simulink model "triplestageSimu"  (R2015a)
settings: Solver=ode45  StartTime=0.0  StopTime=10.0  RelTol=1e-3
values from neighbouring files (symbols this model uses):
  b1 = 0.1    [measfreqresp.m]
  b2 = 0.2    [measfreqresp.m]
  b3 = 0.1    [measfreqresp.m]
  b4 = 0.1    [measfreqresp.m]
libraries: fl_lib x21, nesl_utility x7
settings Model: Creator=Jinwen  LastModifiedBy=Jinwen

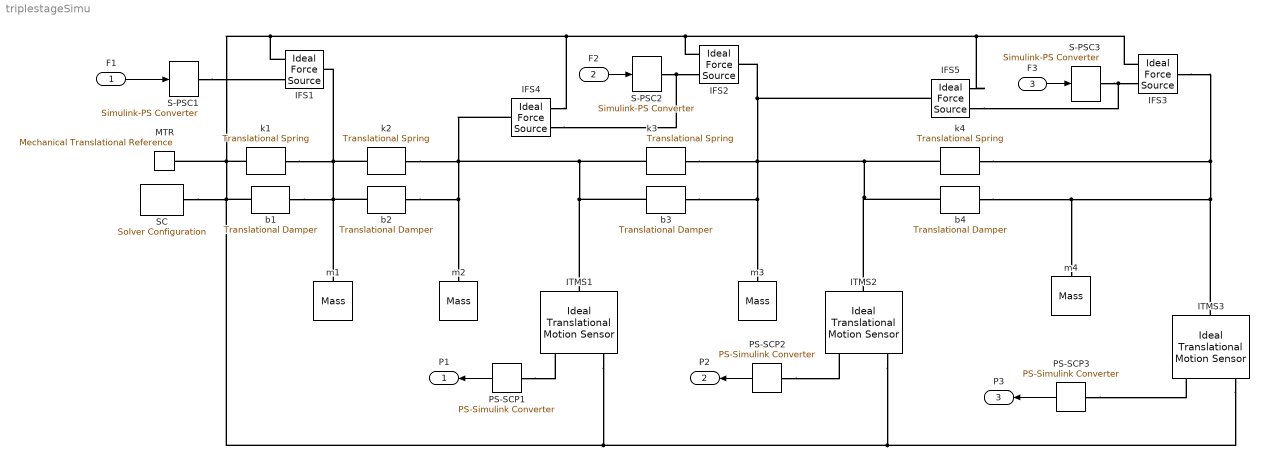
== system triplestageSimu ==
  F1 : Inport
  F2 : Inport  Port=2
  F3 : Inport  Port=3
  IFS{1..5} (5 alike) : fl_lib/Mechanical/Mechanical Sources/Ideal Force Source
  ITMS1 : fl_lib/Mechanical/Mechanical Sensors/Ideal Translational Motion Sensor  offset=0 m
  ITMS2 : fl_lib/Mechanical/Mechanical Sensors/Ideal Translational Motion Sensor  offset=0 m
  ITMS3 : fl_lib/Mechanical/Mechanical Sensors/Ideal Translational Motion Sensor  offset=0 m
  MTR : fl_lib/Mechanical/Translational Elements/Mechanical Translational Reference
  PS-SCP1 : nesl_utility/PS-Simulink Converter  PhysicalDomain=network_engine_domain  SubClassName=ps_output  LeftPortType=input  RightPortType=output  PseudoPeriodic=off  Frequencies=[]  Unit=1  AffineConversion=off
  PS-SCP2 : nesl_utility/PS-Simulink Converter  PhysicalDomain=network_engine_domain  SubClassName=ps_output  LeftPortType=input  RightPortType=output  PseudoPeriodic=off  Frequencies=[]  Unit=1  AffineConversion=off
  PS-SCP3 : nesl_utility/PS-Simulink Converter  PhysicalDomain=network_engine_domain  SubClassName=ps_output  LeftPortType=input  RightPortType=output  PseudoPeriodic=off  Frequencies=[]  Unit=1  AffineConversion=off
  S-PSC1 : nesl_utility/Simulink-PS Converter  PhysicalDomain=network_engine_domain  SubClassName=ps_input  LeftPortType=input  RightPortType=output  PseudoPeriodic=off  Frequencies=[]  NoiseDistribution=none  NoiseParameters=[]  Unit=1  AffineConversion=off  InputFiltering=off  SimscapeFilterOrder=1  InputFilterTimeConstant=0.001  UdotUserProvided=1
  S-PSC2 : nesl_utility/Simulink-PS Converter  PhysicalDomain=network_engine_domain  SubClassName=ps_input  LeftPortType=input  RightPortType=output  PseudoPeriodic=off  Frequencies=[]  NoiseDistribution=none  NoiseParameters=[]  Unit=1  AffineConversion=off  InputFiltering=off  SimscapeFilterOrder=1  InputFilterTimeConstant=0.001  UdotUserProvided=1
  S-PSC3 : nesl_utility/Simulink-PS Converter  PhysicalDomain=network_engine_domain  SubClassName=ps_input  LeftPortType=input  RightPortType=output  PseudoPeriodic=off  Frequencies=[]  NoiseDistribution=none  NoiseParameters=[]  Unit=1  AffineConversion=off  InputFiltering=off  SimscapeFilterOrder=1  InputFilterTimeConstant=0.001  UdotUserProvided=1
  SC : nesl_utility/Solver Configuration  PhysicalDomain=network_engine_domain  SubClassName=solver  LeftPortType=input  RightPortType=generic  Accelerate=off  Tones=[]  Harmonics=[]  SimulateNoise=off  Profile=off  UseLocalSampling=off  EnableSwitchedLinearOptims=on  FrequencyDomain=off  UseCCode=off  RelTol=0.001  AbsTol=1e-06  MinStep=1e-09  ToWorkspace=off  RevertToSquareIcSolve=off  NumHomotopyIterations=100  DoDC=off  ResidualTolerance=1e-09  UseLocalSolver=off  LocalSolverChoice=NE_BACKWARD_EULER_ADVANCER  LocalSolverSampleTime=0.001  DoFixedCost=off  MaxNonlinIter=3  MaxModeIter=2  LinearAlgebra=Sparse  DelaysMemoryBudget=1024  AutomaticFiltering=on  FilteringTimeConstant=0.001
  b1 : fl_lib/Mechanical/Translational Elements/Translational Damper  D=b1 N/(m/s)  v_specify=off  v_priority=High  v=0 m/s  f_specify=off  f_priority=High  f=0 N
  b2 : fl_lib/Mechanical/Translational Elements/Translational Damper  D=b2 N/(m/s)  v_specify=off  v_priority=High  v=0 m/s  f_specify=off  f_priority=High  f=0 N
  b3 : fl_lib/Mechanical/Translational Elements/Translational Damper  D=b3 N/(m/s)  v_specify=off  v_priority=High  v=0 m/s  f_specify=off  f_priority=High  f=0 N
  b4 : fl_lib/Mechanical/Translational Elements/Translational Damper  D=b4 N/(m/s)  v_specify=off  v_priority=High  v=0 m/s  f_specify=off  f_priority=High  f=0 N
  k1 : fl_lib/Mechanical/Translational Elements/Translational Spring  spr_rate=k1 N/m  v_specify=off  v_priority=High  v=0 m/s  f_specify=off  f_priority=High  f=0 N  x_specify=off  x_priority=High  x=0 m
  k2 : fl_lib/Mechanical/Translational Elements/Translational Spring  spr_rate=k2 N/m  v_specify=off  v_priority=High  v=0 m/s  f_specify=off  f_priority=High  f=0 N  x_specify=off  x_priority=High  x=0 m
  k3 : fl_lib/Mechanical/Translational Elements/Translational Spring  spr_rate=k3 N/m  v_specify=off  v_priority=High  v=0 m/s  f_specify=off  f_priority=High  f=0 N  x_specify=off  x_priority=High  x=0 m
  k4 : fl_lib/Mechanical/Translational Elements/Translational Spring  spr_rate=k4 N/m  v_specify=off  v_priority=High  v=0 m/s  f_specify=off  f_priority=High  f=0 N  x_specify=off  x_priority=High  x=0 m
  m1 : fl_lib/Mechanical/Translational Elements/Mass  mass=m1 kg  v_specify=on  v_priority=High  v=0 m/s  f_specify=on  f_priority=High  f=0 N
  m2 : fl_lib/Mechanical/Translational Elements/Mass  mass=m2 kg  v_specify=on  v_priority=High  v=0 m/s  f_specify=on  f_priority=High  f=0 N
  m3 : fl_lib/Mechanical/Translational Elements/Mass  mass=m3 kg  v_specify=on  v_priority=High  v=0 m/s  f_specify=on  f_priority=High  f=0 N
  m4 : fl_lib/Mechanical/Translational Elements/Mass  mass=m4 kg  v_specify=on  v_priority=High  v=0 m/s  f_specify=on  f_priority=High  f=0 N
  P1 : Outport
  P2 : Outport  Port=2
  P3 : Outport  Port=3
  wires:
  F1/1 -> S-PSC1/1
  PS-SCP1/1 -> P1/1
  PS-SCP2/1 -> P2/1
  F2/1 -> S-PSC2/1
  PS-SCP3/1 -> P3/1
  F3/1 -> S-PSC3/1
  connections:
  b1/RConn1 -- ITMS2/RConn1 -- ITMS3/RConn1 -- ITMS1/RConn1 -- IFS5/RConn2 -- IFS3/RConn2 -- IFS2/RConn2 -- IFS4/RConn2 -- IFS1/RConn2 -- k1/RConn1 -- MTR/LConn1 -- SC/RConn1
  S-PSC1/RConn1 -- IFS1/RConn1
  PS-SCP1/LConn1 -- ITMS1/RConn3
  PS-SCP2/LConn1 -- ITMS2/RConn3
  S-PSC2/RConn1 -- IFS4/RConn1 -- IFS2/RConn1
  k2/LConn1 -- IFS4/LConn1 -- b2/LConn1 -- m2/LConn1 -- k3/RConn1 -- b3/RConn1 -- ITMS1/LConn1
  b4/LConn1 -- IFS3/LConn1 -- k4/LConn1 -- ITMS3/LConn1 -- m4/LConn1
  PS-SCP3/LConn1 -- ITMS3/RConn3
  S-PSC3/RConn1 -- IFS5/RConn1 -- IFS3/RConn1
  k1/LConn1 -- k2/RConn1 -- b2/RConn1 -- m1/LConn1 -- b1/LConn1 -- IFS1/LConn1
  k3/LConn1 -- IFS5/LConn1 -- IFS2/LConn1 -- ITMS2/LConn1 -- b4/RConn1 -- k4/RConn1 -- b3/LConn1 -- m3/LConn1
